simulink model "combinedTxRx_ADIDMA"  (R2017b)
settings: Solver=FixedStepDiscrete  StartTime=0.0  StopTime=10.0  RelTol=1e-3
InitFcn:
  | numHeaderBits = 16;
  | %numPreambleBits = 250;
  | AGCBarkerSymbols = 160+28;
  | EQTrainingSymbols = 250;
  | CRCGeneratorLag = 34; % CRCLen + 2
  | 
  | %% AGC Preamble
  | B13bipolar = [0 0 0 0 0 2 2 0 0 2 0 2];
  | rep = [B13bipolar, B13bipolar(1:4)];
  | AGCBarker = repmat(rep,1,10);
  | % Second preamble part
  | B11bipolar = [0 0 0 2 2 2 0 2  2 0 2];
  | TimingBarker = [B11bipolar,B11bipolar,B11bipolar,B11bipolar(1:6)];
  | PreambleBarkersInts = [AGCBarker, TimingBarker];
  | % Convert integer into their bit representation
  | PreambleBarkersBits = zeros(1,length(PreambleBarkersInts)*2);
  | PreambleBarkersBits(1:2:end) = (PreambleBarkersInts==2);
  | 
  | % Constants
  | % First preamble part
  | B13bipolar = [0 0 0 0 0 2 2 0 0 2 0 2];
  | rep = [B13bipolar, B13bipolar(1:4)];
  | AGCBarker = repmat(rep,1,10);
  | % Second preamble part
  | B11bipolar = [0 0 0 2 2 2 0 2  2 0 2];
  | TimingBarker = [B11bipolar,B11bipolar,B11bipolar(1:6)];
  | PreambleBarkersInts = [AGCBarker, TimingBarker];
  | % Convert integer into their bit representation
  | PreambleBarkersBits = false(1,length(PreambleBarkersInts)*2);
  | PreambleBarkersBits(1:2:end) = logical(PreambleBarkersInts==2);
  | pLen = uint16(length(PreambleBarkersBits));
  | 
  | 
  | %%%%%%%%%%%%%%%%%%%%%%%%%%
  | %% RX
  | %%%%%%%%%%%%%%%%%%%%%%%%%%
  | 
  | barker = comm.BarkerCode('SamplesPerFrame', 28, 'Length', 11);
  | seq = barker()+1;
  | M = 4;
  | hPSKModTrain   = comm.PSKModulator(M, ...
  |     'PhaseOffset',pi/4, ...
  |     'SymbolMapping','Binary');
  | xPreambleSeq = hPSKModTrain(seq);
  | 
  | 
  | %%%%%%%%%%%%
  | 
  | % AGC Preamble
  | reps = 5;
  | barker = comm.BarkerCode('SamplesPerFrame', 16, 'Length', 13);
  | seq = barker()+1;
  | %preamble = zeros(16*reps,1);
  | preambleFull = repmat(seq,reps,1);
  | rctFilt = comm.RaisedCosineTransmitFilter('FilterSpanInSymbols', 128,...
  | 'RolloffFactor',0.5,...
  | 'OutputSamplesPerSymbol',4);
  | preambleFullFilt = rctFilt(preambleFull);
  | 
  | %%%%%%%%%%%%
  | ... (+62 lines)
undefined symbols (not defined in the file or in its folder): j
libraries: simulink x20, dsphdlfiltering x20, hdlsllib x7, dspsigops x4, commseqgen3 x3, commdigbbndpm3 x3, commcrc2 x2, commcnvcod2 x2, commfilt2 x2, commsource2 x1, dspstat3 x1
(part 2 of 3)

== system combinedTxRx_ADIDMA/Combined TX and RX/Receiver HDL/Frame Recover/Equalization and Demodulation/DFE ==
  note: Generate training sequence when barker is found
  Trigger : Inport  PortDimensions=1
  data : Inport  Port=2  PortDimensions=1
      settings: SignalType=complex
  EQmu : Inport  Port=3
  DFE : Subsystem  mask{numFTaps=5, numBTaps=3, mu=0.01, refTap=2}
      mask prompts: numFTaps "Num Forward Taps"; numBTaps "Num Backward Taps"; mu "Step Size"; refTap "Reference Tap"
  Delay data so DFE can reset : Delay  DelayLength=1
  Delay ref so DFE can reset : Delay  DelayLength=1
  Equalizer : MATLAB Function  Commented=on  TreatAsAtomicUnit=on
  PN Sequence Generator : commseqgen3/PN Sequence Generator  poly='z^5 + z^3 + z^1 + 1'  ini_sta=[1 1 1 0 0]  outBitMaskSource=Dialog parameter  shift=0  outVarSiz=off  maxOutSizeMode=Dialog parameter  maxOutSize=[10 1]  Ts=-1  sampPerFrame=1  reset=on  bitPackedOutputs=on  outDataType=Smallest unsigned integer  numPackedBits=2  bitPackDataSigned=off  bitPackedOutDType=Smallest integer
      settings: SourceProductName=Communications System Toolbox
  Packeted To Unpacked : Subsystem
  QPSK Modulator Baseband : commdigbbndpm3/QPSK Modulator Baseband  InType=Bit  Enc=Binary  Ph=pi/4  outDtype=Fixed-point  outWordLen=16  outUDDataType=sfix(16)  outFracLenMode=User-defined  outFracLen=15  outDataTypeStr=fixdt(1,16,15)  outLastDataTypeStr=fixdt(1,16,15)
  Terminator1 : Terminator
  dataEQed : Outport
  start : Outport  Port=2
  wires:
  data/1 -> Delay data so DFE can reset/1
  PN Sequence Generator/1 -> Packeted To Unpacked/1(In1)
  Packeted To Unpacked/1(Out1) -> QPSK Modulator Baseband/1
  QPSK Modulator Baseband/1 -> Delay ref so DFE can reset/1
  DFE/3(start) -> start/1
  Trigger/1 -> DFE/1(reset), PN Sequence Generator/1
  DFE/2(err) -> Terminator1/1
  DFE/1(eqOut) -> dataEQed/1
  Delay data so DFE can reset/1 -> DFE/2(dataIn)
  Delay ref so DFE can reset/1 -> DFE/3(training)
  EQmu/1 -> DFE/4(EQmu)

== system combinedTxRx_ADIDMA/Combined TX and RX/Receiver HDL/Frame Recover/Frequency Recovery/Loop Filter ==
  note: This inflation is necessary
  note: Proportional-plus-Integrator Loop Filter,
      | Infinite DC Response to guarantee convergence
  e : Inport
  Add1 : Sum  RndMeth=Nearest  OutDataTypeStr=Inherit: Same as first input
  Add2 : Sum  OutDataTypeStr=Inherit: Same as first input
  Data Type Conversion : DataTypeConversion  OutDataTypeStr=fixdt(1,25,20)
  Delay : Delay  DelayLength=1
  Delay3 : Delay  DelayLength=1
  Delay4 : Delay  DelayLength=1
  K1 : Gain  Gain=K2  OutDataTypeStr=Inherit: Same as input
  K2 : Gain  Gain=K1  OutDataTypeStr=Inherit: Same as input
  Sum2 : Sum  OutDataTypeStr=Inherit: Same as first input
  v : Outport
  wires:
  K1/1 -> Sum2/1
  Add1/1 -> Sum2/2
  e/1 -> K2/1, K1/1
  K2/1 -> Delay/1, Add1/2
  Delay/1 -> Add1/1
  Sum2/1 -> Delay3/1
  Delay3/1 -> Add2/1
  Delay4/1 -> Add2/2
  Add2/1 -> Delay4/1, Data Type Conversion/1
  Data Type Conversion/1 -> v/1

== system combinedTxRx_ADIDMA/Combined TX and RX/Receiver HDL/Frame Recover/Frequency Recovery/Loop Filter Configurable ==
  note: This inflation is necessary
  note: Proportional-plus-Integrator Loop Filter,
      | Infinite DC Response to guarantee convergence
  e : Inport
  LoopBW : Inport  Port=2
  Add1 : Sum  RndMeth=Nearest  OutDataTypeStr=Inherit: Same as first input
  Add2 : Sum  OutDataTypeStr=Inherit: Same as first input
  Data Type Conversion : DataTypeConversion  OutDataTypeStr=fixdt(1,25,20)
  Delay : Delay  DelayLength=1
  Delay3 : Delay  DelayLength=1
  Delay4 : Delay  DelayLength=1
  Direct Lookup Table (n-D) : LookupNDDirect  NumberOfTableDimensions=1  Table=K1  DiagnosticForOutOfRangeInput=Error
  Direct Lookup Table (n-D)1 : LookupNDDirect  NumberOfTableDimensions=1  Table=K2  DiagnosticForOutOfRangeInput=Error
  Product : Product  OutDataTypeStr=Inherit: Same as first input
  Product1 : Product  OutDataTypeStr=Inherit: Same as first input
  Sum2 : Sum  OutDataTypeStr=Inherit: Same as first input
  v : Outport
  wires:
  Product/1 -> Sum2/1
  Add1/1 -> Sum2/2
  e/1 -> Product1/1, Product/1
  Product1/1 -> Delay/1, Add1/2
  Delay/1 -> Add1/1
  Sum2/1 -> Delay3/1
  Delay3/1 -> Add2/1
  Delay4/1 -> Add2/2
  Add2/1 -> Delay4/1, Data Type Conversion/1
  Data Type Conversion/1 -> v/1
  Direct Lookup Table (n-D)/1 -> Product/2
  Direct Lookup Table (n-D)1/1 -> Product1/2
  LoopBW/1 -> Direct Lookup Table (n-D)/1, Direct Lookup Table (n-D)1/1

== system combinedTxRx_ADIDMA/Combined TX and RX/Receiver HDL/Frame Recover/Frequency Recovery/Phase Shift FP ==
  note: Sign Comes from original
      | loop filter design
  In1 : Inport
  Phi : Inport  Port=2
  Cosine HDL Optimized : hdlsllib/Lookup Tables/Cosine HDL Optimized  OutputFormula=exp(j*2*pi*u)  NumDataPoints=256  TableDataTypeStr=fixdt(0,31,20)  SimulateLUTROMDelay=off
      settings: SourceProductName=HDL Coder  SourceProductBaseCode=HD
  Gain : Gain  Gain=-1/(2*pi)  ParamDataTypeStr=fixdt(1,25,20)  OutDataTypeStr=fixdt(1,16,12)  SaturateOnIntegerOverflow=on
  Product : Product  OutDataTypeStr=fixdt(1,16,13)  SaturateOnIntegerOverflow=on
  Out1 : Outport
  wires:
  Product/1 -> Out1/1
  Cosine HDL Optimized/1 -> Product/2
  In1/1 -> Product/1
  Phi/1 -> Gain/1
  Gain/1 -> Cosine HDL Optimized/1

== system combinedTxRx_ADIDMA/Combined TX and RX/Receiver HDL/Frame Recover/Gardner Timing Recovery/Gardner TED Blocks ==
  note: An input of 4 should not
      | happen unless the input is all zeros
  note: This is for QPSK and 4 SamplesPerSymbol ONLY
  data : Inport
  strobe : Inport  Port=2
  Add : Sum  OutDataTypeStr=fixdt(1,16,15)
  Check Only Strobe Condition : simulink/Logic and Bit Operations/Compare To Constant  relop===  const=uint8(1)  OutDataTypeStr=boolean
  Complex to Real-Imag : ComplexToRealImag
  Constant : Constant  Value=0  OutDataTypeStr=Inherit: Inherit via back propagation  SampleTime=-1
  Display : Display
  Imag Error : Subsystem
  Logical Operator : Logic  AllPortsSameDT=off  OutDataTypeStr=boolean
  Map [0,1,2,3,4] to [0,1,2,2,2] : LookupNDDirect  NumberOfTableDimensions=1  Table=[0 1 2 2 2]  DiagnosticForOutOfRangeInput=Error  TableDataTypeStr=uint8
  Real Error : Subsystem
  Strobe Buffer1 : simulink/Discrete/Tapped Delay  vinit=0.0  samptime=-1  NumDelays=samplesPerSymbol-1  DelayOrder=Oldest  includeCurrent=on
  Sum of Elements1 : Sum  Inputs=+  OutDataTypeStr=int8
  Switch : Switch  Criteria=u2 ~= 0  SaturateOnIntegerOverflow=on
  e : Outport
  wires:
  Switch/1 -> e/1
  strobe/1 -> Strobe Buffer1/1, Logical Operator/2
  Complex to Real-Imag/2 -> Imag Error/1(data)
  Sum of Elements1/1 -> Display/1, Check Only Strobe Condition/1, Map [0,1,2,3,4] to [0,1,2,2,2]/1
  Check Only Strobe Condition/1 -> Logical Operator/1
  Constant/1 -> Switch/3
  Complex to Real-Imag/1 -> Real Error/1(data)
  data/1 -> Complex to Real-Imag/1
  Map [0,1,2,3,4] to [0,1,2,2,2]/1 -> Imag Error/2(strobe sum), Real Error/2(strobe sum)
  Strobe Buffer1/1 -> Sum of Elements1/1
  Real Error/1(Out1) -> Add/1
  Imag Error/1(Out1) -> Add/2
  Add/1 -> Switch/1
  Logical Operator/1 -> Switch/2

== system combinedTxRx_ADIDMA/Combined TX and RX/Receiver HDL/Frame Recover/Gardner Timing Recovery/InterpControl_Blocks1 ==
  note: e<<1/SPS
  note: Mu is always positive
  e : Inport
  1/SPS1 : Constant  Value=fi(1/samplesPerSymbol,0,2,2)  OutDataTypeStr=fixdt(0,2,2)  SampleTime=-1
  Add1 : Sum  OutDataTypeStr=fixdt(0,16,16)
  Calculate New mu : Subsystem
  Display{,1..3} (4 alike) : Display
  Mod 1 : Subsystem
  NCOCounter State : Delay  DelayLength=1  InitialCondition=0
  Subtract1 : Sum  Inputs=-+  OutDataTypeStr=Inherit: Same as first input
  Update mu on strobe : Switch  Criteria=u2 > Threshold
  saved mu : Delay  DelayLength=1
  strobe == W>NCOCounter : RelationalOperator  Operator=>  OutDataTypeStr=boolean  RndMeth=Nearest
  strobe : Outport
  mu : Outport  Port=2
  wires:
  strobe == W>NCOCounter/1 -> Update mu on strobe/2, strobe/1
  Update mu on strobe/1 -> Display3/1, mu/1, saved mu/1
  saved mu/1 -> Update mu on strobe/3
  Calculate New mu/1(mu) -> Display/1, Update mu on strobe/1
  e/1 -> Add1/1
  NCOCounter State/1 -> Subtract1/2, Display1/1, strobe == W>NCOCounter/2, Calculate New mu/2(NCOCounter)
  Subtract1/1 -> Mod 1/1(In1)
  Mod 1/1(Out1) -> NCOCounter State/1
  1/SPS1/1 -> Add1/2
  Add1/1 -> Calculate New mu/1(W), strobe == W>NCOCounter/1, Display2/1, Subtract1/1

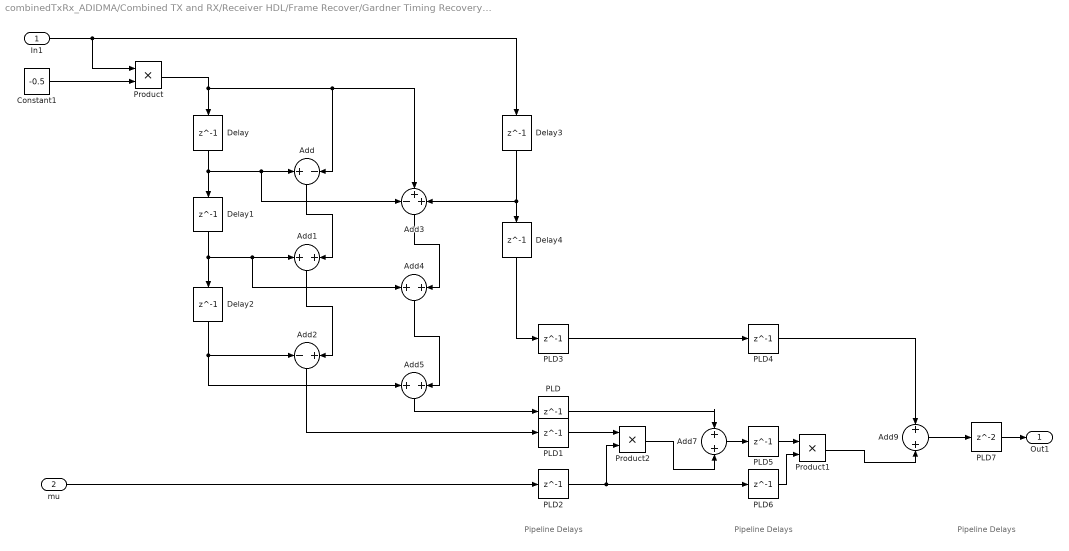
== system combinedTxRx_ADIDMA/Combined TX and RX/Receiver HDL/Frame Recover/Gardner Timing Recovery/Interpolator ==
  note: Pipeline Delays
  note: Pipeline Delays
  note: Pipeline Delays
  In1 : Inport
  mu : Inport  Port=2
  Add : Sum  Inputs=+-  OutDataTypeStr=Inherit: Same as first input
  Add{1,4..5,7} (4 alike) : Sum
  Add2 : Sum  Inputs=-+
  Add3 : Sum  Inputs=-++
  Add9 : Sum  OutDataTypeStr=fixdt(1,16,10)
  Constant1 : Constant  Value=-0.5  OutDataTypeStr=fixdt(1,2,2)  SampleTime=-1
  Delay{,1..4} (5 alike) : Delay  DelayLength=1
  PLD{,1..6} (7 alike) : Delay  DelayLength=1
  PLD7 : Delay
  Product : Product  OutDataTypeStr=fixdt(1,16,14)
  Product1 : Product
  Product2 : Product  OutDataTypeStr=fixdt(1,16,10)
  Out1 : Outport
  wires:
  In1/1 -> Delay3/1, Product/1
  Product/1 -> Add3/2, Add/2, Delay/1
  Delay/1 -> Add3/1, Add/1, Delay1/1
  Delay1/1 -> Add4/1, Add1/1, Delay2/1
  Add/1 -> Add1/2
  Delay2/1 -> Add5/1, Add2/1
  Add1/1 -> Add2/2
  Add3/1 -> Add4/2
  Add4/1 -> Add5/2
  Add2/1 -> PLD1/1
  mu/1 -> PLD2/1
  Add5/1 -> PLD/1
  Product2/1 -> Add7/2
  Add9/1 -> PLD7/1
  Delay3/1 -> Delay4/1, Add3/3
  Delay4/1 -> PLD3/1
  Add7/1 -> PLD5/1
  Product1/1 -> Add9/2
  Constant1/1 -> Product/2
  PLD/1 -> Add7/1
  PLD1/1 -> Product2/1
  PLD2/1 -> Product2/2, PLD6/1
  PLD3/1 -> PLD4/1
  PLD4/1 -> Add9/1
  PLD5/1 -> Product1/1
  PLD6/1 -> Product1/2
  PLD7/1 -> Out1/1

== system combinedTxRx_ADIDMA/Combined TX and RX/Receiver HDL/Frame Recover/Gardner Timing Recovery/LoopFilter1 ==
  e : Inport
  Delay1 : Delay  DelayLength=1
  Delay2 : Delay  DelayLength=1
  Proportional Gain : Gain  Gain=fi(ProportionalGain,1,16,15)  OutDataTypeStr=fixdt(1,16,24)
  v : Outport
  wires:
  e/1 -> Delay2/1
  Proportional Gain/1 -> Delay1/1
  Delay2/1 -> Proportional Gain/1
  Delay1/1 -> v/1

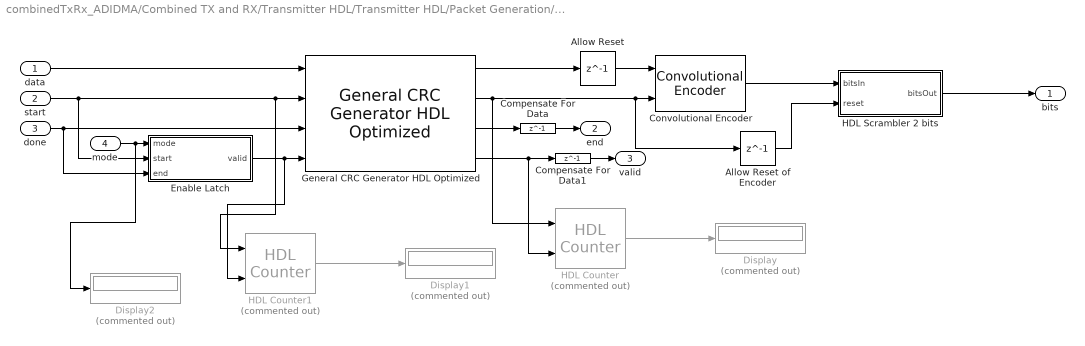
== system combinedTxRx_ADIDMA/Combined TX and RX/Transmitter HDL/Transmitter HDL/Packet Generation/Payload ==
  data : Inport
  start : Inport  Port=2
  done : Inport  Port=3
  mode : Inport  Port=4
  Allow Reset : Delay  DelayLength=1
  Allow Reset of Encoder : Delay  DelayLength=1
  Compensate For Data : Delay  DelayLength=1
  Compensate For Data1 : Delay  DelayLength=1
  Convolutional Encoder : commcnvcod2/Convolutional Encoder  trellis=poly2trellis(7, [171 133])  opMode=Reset on nonzero input via port  DelayedResetAction=on  hasIniStPort=off  hasFinStPort=off  usePuncVector=off  punctureVector=[1; 1; 0; 1; 0; 1]  reset=Unused parameter value
      settings: SourceProductName=Communications System Toolbox  SourceProductBaseCode=CM
  Display : Display  Commented=on
  Display1 : Display  Commented=on
  Display2 : Display  Commented=on
  Enable Latch : Subsystem
  General CRC Generator HDL Optimized : commcrc2/General CRC Generator HDL Optimized  Polynomial=[1 0 0 0 0 0 1 0 0 1 1 0 0 0 0 0 1 0 0 0 1 1 1 0 1 1 0 1 1 0 1 1 1]  InitialState=0  DirectMethod=off  ReflectInput=off  ReflectCRCChecksum=off  FinalXORValue=0  SimulateUsing=Code generation
      settings: SourceProductName=Communications System Toolbox  SourceProductBaseCode=CM
  HDL Counter : hdlsllib/Sources/HDL Counter  Commented=on  CountType=Count limited  CountInit=0  CountStep=1  CountMax=1e4  CountFromType=Initial value  CountFrom=0  CountResetPort=on  CountLoadPort=off  CountEnbPort=on  CountDirPort=off  CountDataType=Unsigned  CountWordLen=16  CountFracLen=0  CountSampTime=1
      settings: SourceProductBaseCode=HD
  HDL Counter1 : hdlsllib/Sources/HDL Counter  Commented=on  CountType=Count limited  CountInit=0  CountStep=1  CountMax=1e4  CountFromType=Initial value  CountFrom=0  CountResetPort=on  CountLoadPort=off  CountEnbPort=on  CountDirPort=off  CountDataType=Unsigned  CountWordLen=16  CountFracLen=0  CountSampTime=1
      settings: SourceProductBaseCode=HD
  HDL Scrambler 2 bits : Subsystem  mask{poly=[1 1 0 1 0 1 0 1], init_state=[0 1 0 0 0 1 0]}
      mask prompts: poly "Polynomial"; init_state "Initial State"
  bits : Outport
  end : Outport  Port=2
  valid : Outport  Port=3
  wires:
  General CRC Generator HDL Optimized/1 -> Allow Reset/1
  data/1 -> General CRC Generator HDL Optimized/1
  start/1 -> Enable Latch/2(start), HDL Counter1/1, General CRC Generator HDL Optimized/2
  General CRC Generator HDL Optimized/4 -> HDL Counter/2, Compensate For Data1/1
  done/1 -> Enable Latch/3(end), General CRC Generator HDL Optimized/3
  mode/1 -> Display2/1, Enable Latch/1(mode)
  Convolutional Encoder/1 -> HDL Scrambler 2 bits/1(bitsIn)
  General CRC Generator HDL Optimized/2 -> HDL Counter/1, Allow Reset of Encoder/1, Convolutional Encoder/2
  HDL Scrambler 2 bits/1(bitsOut) -> bits/1
  Enable Latch/1(valid) -> HDL Counter1/2, General CRC Generator HDL Optimized/4
  Allow Reset/1 -> Convolutional Encoder/1
  Allow Reset of Encoder/1 -> HDL Scrambler 2 bits/2(reset)
  HDL Counter/1 -> Display/1
  HDL Counter1/1 -> Display1/1
  Compensate For Data/1 -> end/1
  Compensate For Data1/1 -> valid/1
  General CRC Generator HDL Optimized/3 -> Compensate For Data/1

== system combinedTxRx_ADIDMA/Combined TX and RX/Transmitter HDL/Transmitter HDL/Packet Generation/Preamble ==
  reset : Inport
  Barker Even : LookupNDDirect  NumberOfTableDimensions=1  Table=[PreambleBarkersBits(4:2:end),false(1,400)]  DiagnosticForOutOfRangeInput=Error  TableDataTypeStr=boolean
  Barker Odd : LookupNDDirect  NumberOfTableDimensions=1  Table=[PreambleBarkersBits(3:2:end-1),false(1,400)]  DiagnosticForOutOfRangeInput=Error  TableDataTypeStr=boolean
  Delay{,1..3} (4 alike) : Delay  DelayLength=1
  Enable at end of barker : simulink/Logic and Bit Operations/Compare To Constant  relop=<  const=pLen/2-1  OutDataTypeStr=boolean
  HDL Counter : hdlsllib/Sources/HDL Counter  CountType=Count limited  CountInit=0  CountStep=1  CountMax=pLen/2-2+400  CountFromType=Initial value  CountFrom=0  CountResetPort=on  CountLoadPort=off  CountEnbPort=off  CountDirPort=off  CountDataType=Unsigned  CountWordLen=16  CountFracLen=0  CountSampTime=1
      settings: SourceProductBaseCode=HD
  PN Sequence For EQ : commseqgen3/PN Sequence Generator  poly='z^5 + z^3 + z^1 + 1'  ini_sta=[1 1 1 0 0]  outBitMaskSource=Dialog parameter  shift=0  outVarSiz=off  maxOutSizeMode=Dialog parameter  maxOutSize=[10 1]  Ts=-1  sampPerFrame=1  reset=on  bitPackedOutputs=on  outDataType=double  numPackedBits=2  bitPackDataSigned=off  bitPackedOutDType=Smallest integer
      settings: SourceProductName=Communications System Toolbox
  Reset When Barkers Are Done : simulink/Logic and Bit Operations/Compare To Constant  relop===  const=pLen/2-1  OutDataTypeStr=boolean
  Switch1 : Switch  Threshold=1
  Unpack1 : Subsystem
  Vector Concatenate1 : Concatenate
  Out1 : Outport
  wires:
  reset/1 -> HDL Counter/1
  Barker Odd/1 -> Vector Concatenate1/1
  Barker Even/1 -> Vector Concatenate1/2
  PN Sequence For EQ/1 -> Unpack1/1(In1)
  Switch1/1 -> Out1/1
  Reset When Barkers Are Done/1 -> PN Sequence For EQ/1
  HDL Counter/1 -> Delay/1
  Delay/1 -> Enable at end of barker/1, Reset When Barkers Are Done/1, Barker Even/1, Barker Odd/1
  Vector Concatenate1/1 -> Delay1/1
  Enable at end of barker/1 -> Delay2/1
  Unpack1/1(Out1) -> Delay3/1
  Delay1/1 -> Switch1/1
  Delay2/1 -> Switch1/2
  Delay3/1 -> Switch1/3

== system combinedTxRx_ADIDMA/Combined TX and RX/Transmitter HDL/Transmitter HDL/Packet Generation/Random Data ==
  In1 : Inport
  Random Data Gen : commseqgen3/PN Sequence Generator  poly='z^3 + z^2 + 1'  ini_sta=[0 0 1]  outBitMaskSource=Dialog parameter  shift=0  outVarSiz=off  maxOutSizeMode=Dialog parameter  maxOutSize=[10 1]  Ts=-1  sampPerFrame=1  reset=on  bitPackedOutputs=on  outDataType=double  numPackedBits=2  bitPackDataSigned=off  bitPackedOutDType=Smallest integer
      settings: SourceProductName=Communications System Toolbox
  Unpack : Subsystem
  Out1 : Outport
  wires:
  In1/1 -> Random Data Gen/1
  Unpack/1(Out1) -> Out1/1
  Random Data Gen/1 -> Unpack/1(In1)

== system combinedTxRx_ADIDMA/Combined TX and RX/Receiver HDL/Frame Recover/Barker Locate/Measure Phase Ambiguity/Find Max and Set Output Shift ==
  In1 : Inport
  In2 : Inport  Port=2
  In4 : Inport  Port=3
  In5 : Inport  Port=4
  Enable : EnablePort
  Complex to Real-Imag{,1..3} (4 alike) : ComplexToRealImag  Output=Imag
  Direct Lookup Table (n-D) : LookupNDDirect  NumberOfTableDimensions=1  Table=exp(-(0:pi/2:(pi*3/2)) .* 1i).'  DiagnosticForOutOfRangeInput=Error  TableDataTypeStr=fixdt(1,16,13)
  Display : Display
  Display1 : Display
  Maximum : dspstat3/Maximum  operation=maximum  fcn=Index  indexBase=Zero  operateOver=Each column  Dimension=1  InputProcessing=Columns as channels (frame based)  reset=None  roiEnable=off  roiType=Rectangles  roiPortion=Entire ROI  roiOutput=Individual statistics for each ROI  roiFlag=off  roundingMode=Floor  overflowMode=off  accumDataTypeStr=Inherit: Same as product output  accumLastDataTypeStr=Inherit: Same as product output
  Vector Concatenate : Concatenate  NumInputs=4
  Vector Concatenate1 : Concatenate  NumInputs=4
  Out1 : Outport  InitialOutput=0
  wires:
  Direct Lookup Table (n-D)/1 -> Out1/1
  In4/1 -> Vector Concatenate1/3, Complex to Real-Imag2/1
  In2/1 -> Vector Concatenate1/2, Complex to Real-Imag1/1
  In5/1 -> Vector Concatenate1/4, Complex to Real-Imag3/1
  In1/1 -> Vector Concatenate1/1, Complex to Real-Imag/1
  Maximum/1 -> Direct Lookup Table (n-D)/1
  Vector Concatenate/1 -> Display/1, Maximum/1
  Vector Concatenate1/1 -> Display1/1
  Complex to Real-Imag1/1 -> Vector Concatenate/2
  Complex to Real-Imag3/1 -> Vector Concatenate/4
  Complex to Real-Imag2/1 -> Vector Concatenate/3
  Complex to Real-Imag/1 -> Vector Concatenate/1

== system combinedTxRx_ADIDMA/Combined TX and RX/Receiver HDL/Frame Recover/Barker Locate/Measure Phase Ambiguity/HDL Opt Complex FIR4 ==
  In1 : Inport
  validIn : Inport  Port=2
  Add : Sum  Inputs=+-  AccumDataTypeStr=fixdt(1,16,0)
  Complex to Real-Imag : ComplexToRealImag
  Discrete FIR Filter HDL Optimized : dsphdlfiltering/Discrete FIR Filter HDL Optimized  Numerator=real(Taps)  Sharing=off  SharingFactor=2  SimulateUsing=Code generation  roundingMode=Floor  overflowMode=off  CoefficientsDataTypeStr=Inherit: Same word length as input  CoefficientsMin=[]  CoefficientsMax=[]  OutputDataTypeStr=fixdt(1,16,0)  OutputMin=[]  OutputMax=[]  ValidInPort=on  ReadyPort=off
      settings: SourceProductName=DSP System Toolbox  SourceProductBaseCode=DS
  Discrete FIR Filter HDL Optimized1 : dsphdlfiltering/Discrete FIR Filter HDL Optimized  Numerator=imag(Taps)  Sharing=off  SharingFactor=2  SimulateUsing=Code generation  roundingMode=Floor  overflowMode=off  CoefficientsDataTypeStr=Inherit: Same word length as input  CoefficientsMin=[]  CoefficientsMax=[]  OutputDataTypeStr=fixdt(1,16,0)  OutputMin=[]  OutputMax=[]  ValidInPort=on  ReadyPort=off
      settings: SourceProductName=DSP System Toolbox  SourceProductBaseCode=DS
  Discrete FIR Filter HDL Optimized2 : dsphdlfiltering/Discrete FIR Filter HDL Optimized  Numerator=real(Taps)  Sharing=off  SharingFactor=2  SimulateUsing=Code generation  roundingMode=Floor  overflowMode=off  CoefficientsDataTypeStr=Inherit: Same word length as input  CoefficientsMin=[]  CoefficientsMax=[]  OutputDataTypeStr=fixdt(1,16,0)  OutputMin=[]  OutputMax=[]  ValidInPort=on  ReadyPort=off
      settings: SourceProductName=DSP System Toolbox  SourceProductBaseCode=DS
  Discrete FIR Filter HDL Optimized3 : dsphdlfiltering/Discrete FIR Filter HDL Optimized  Numerator=imag(Taps)  Sharing=off  SharingFactor=2  SimulateUsing=Code generation  roundingMode=Floor  overflowMode=off  CoefficientsDataTypeStr=Inherit: Same word length as input  CoefficientsMin=[]  CoefficientsMax=[]  OutputDataTypeStr=fixdt(1,16,0)  OutputMin=[]  OutputMax=[]  ValidInPort=on  ReadyPort=off
      settings: SourceProductName=DSP System Toolbox  SourceProductBaseCode=DS
  Logical Operator : Logic  Inputs=4  AllPortsSameDT=off  OutDataTypeStr=boolean
  Real-Imag to Complex : RealImagToComplex
  Subtract : Sum  OutDataTypeStr=int16
  Out1 : Outport
  validOut : Outport  Port=2
  wires:
  Discrete FIR Filter HDL Optimized/1 -> Add/1
  Logical Operator/1 -> validOut/1
  Discrete FIR Filter HDL Optimized/2 -> Logical Operator/1
  Discrete FIR Filter HDL Optimized1/2 -> Logical Operator/2
  Discrete FIR Filter HDL Optimized1/1 -> Add/2
  validIn/1 -> Discrete FIR Filter HDL Optimized3/2, Discrete FIR Filter HDL Optimized2/2, Discrete FIR Filter HDL Optimized1/2, Discrete FIR Filter HDL Optimized/2
  In1/1 -> Complex to Real-Imag/1
  Complex to Real-Imag/1 -> Discrete FIR Filter HDL Optimized3/1, Discrete FIR Filter HDL Optimized/1
  Discrete FIR Filter HDL Optimized2/2 -> Logical Operator/3
  Discrete FIR Filter HDL Optimized3/2 -> Logical Operator/4
  Complex to Real-Imag/2 -> Discrete FIR Filter HDL Optimized2/1, Discrete FIR Filter HDL Optimized1/1
  Discrete FIR Filter HDL Optimized2/1 -> Subtract/1
  Discrete FIR Filter HDL Optimized3/1 -> Subtract/2
  Real-Imag to Complex/1 -> Out1/1
  Subtract/1 -> Real-Imag to Complex/2
  Add/1 -> Real-Imag to Complex/1

== system combinedTxRx_ADIDMA/Combined TX and RX/Receiver HDL/Frame Recover/Barker Locate/Measure Phase Ambiguity/HDL Opt Complex FIR5 ==
  In1 : Inport
  validIn : Inport  Port=2
  Add : Sum  Inputs=+-  AccumDataTypeStr=fixdt(1,16,0)
  Complex to Real-Imag : ComplexToRealImag
  Discrete FIR Filter HDL Optimized : dsphdlfiltering/Discrete FIR Filter HDL Optimized  Numerator=real(Taps)  Sharing=off  SharingFactor=2  SimulateUsing=Code generation  roundingMode=Floor  overflowMode=off  CoefficientsDataTypeStr=Inherit: Same word length as input  CoefficientsMin=[]  CoefficientsMax=[]  OutputDataTypeStr=fixdt(1,16,0)  OutputMin=[]  OutputMax=[]  ValidInPort=on  ReadyPort=off
      settings: SourceProductName=DSP System Toolbox  SourceProductBaseCode=DS
  Discrete FIR Filter HDL Optimized1 : dsphdlfiltering/Discrete FIR Filter HDL Optimized  Numerator=imag(Taps)  Sharing=off  SharingFactor=2  SimulateUsing=Code generation  roundingMode=Floor  overflowMode=off  CoefficientsDataTypeStr=Inherit: Same word length as input  CoefficientsMin=[]  CoefficientsMax=[]  OutputDataTypeStr=fixdt(1,16,0)  OutputMin=[]  OutputMax=[]  ValidInPort=on  ReadyPort=off
      settings: SourceProductName=DSP System Toolbox  SourceProductBaseCode=DS
  Discrete FIR Filter HDL Optimized2 : dsphdlfiltering/Discrete FIR Filter HDL Optimized  Numerator=real(Taps)  Sharing=off  SharingFactor=2  SimulateUsing=Code generation  roundingMode=Floor  overflowMode=off  CoefficientsDataTypeStr=Inherit: Same word length as input  CoefficientsMin=[]  CoefficientsMax=[]  OutputDataTypeStr=fixdt(1,16,0)  OutputMin=[]  OutputMax=[]  ValidInPort=on  ReadyPort=off
      settings: SourceProductName=DSP System Toolbox  SourceProductBaseCode=DS
  Discrete FIR Filter HDL Optimized3 : dsphdlfiltering/Discrete FIR Filter HDL Optimized  Numerator=imag(Taps)  Sharing=off  SharingFactor=2  SimulateUsing=Code generation  roundingMode=Floor  overflowMode=off  CoefficientsDataTypeStr=Inherit: Same word length as input  CoefficientsMin=[]  CoefficientsMax=[]  OutputDataTypeStr=fixdt(1,16,0)  OutputMin=[]  OutputMax=[]  ValidInPort=on  ReadyPort=off
      settings: SourceProductName=DSP System Toolbox  SourceProductBaseCode=DS
  Logical Operator : Logic  Inputs=4  AllPortsSameDT=off  OutDataTypeStr=boolean
  Real-Imag to Complex : RealImagToComplex
  Subtract : Sum  OutDataTypeStr=int16
  Out1 : Outport
  validOut : Outport  Port=2
  wires:
  Discrete FIR Filter HDL Optimized/1 -> Add/1
  Logical Operator/1 -> validOut/1
  Discrete FIR Filter HDL Optimized/2 -> Logical Operator/1
  Discrete FIR Filter HDL Optimized1/2 -> Logical Operator/2
  Discrete FIR Filter HDL Optimized1/1 -> Add/2
  validIn/1 -> Discrete FIR Filter HDL Optimized3/2, Discrete FIR Filter HDL Optimized2/2, Discrete FIR Filter HDL Optimized1/2, Discrete FIR Filter HDL Optimized/2
  In1/1 -> Complex to Real-Imag/1
  Complex to Real-Imag/1 -> Discrete FIR Filter HDL Optimized3/1, Discrete FIR Filter HDL Optimized/1
  Discrete FIR Filter HDL Optimized2/2 -> Logical Operator/3
  Discrete FIR Filter HDL Optimized3/2 -> Logical Operator/4
  Complex to Real-Imag/2 -> Discrete FIR Filter HDL Optimized2/1, Discrete FIR Filter HDL Optimized1/1
  Discrete FIR Filter HDL Optimized2/1 -> Subtract/1
  Discrete FIR Filter HDL Optimized3/1 -> Subtract/2
  Real-Imag to Complex/1 -> Out1/1
  Subtract/1 -> Real-Imag to Complex/2
  Add/1 -> Real-Imag to Complex/1

== system combinedTxRx_ADIDMA/Combined TX and RX/Receiver HDL/Frame Recover/Barker Locate/Measure Phase Ambiguity/HDL Opt Complex FIR6 ==
  In1 : Inport
  validIn : Inport  Port=2
  Add : Sum  Inputs=+-  AccumDataTypeStr=fixdt(1,16,0)
  Complex to Real-Imag : ComplexToRealImag
  Discrete FIR Filter HDL Optimized : dsphdlfiltering/Discrete FIR Filter HDL Optimized  Numerator=real(Taps)  Sharing=off  SharingFactor=2  SimulateUsing=Code generation  roundingMode=Floor  overflowMode=off  CoefficientsDataTypeStr=Inherit: Same word length as input  CoefficientsMin=[]  CoefficientsMax=[]  OutputDataTypeStr=fixdt(1,16,0)  OutputMin=[]  OutputMax=[]  ValidInPort=on  ReadyPort=off
      settings: SourceProductName=DSP System Toolbox  SourceProductBaseCode=DS
  Discrete FIR Filter HDL Optimized1 : dsphdlfiltering/Discrete FIR Filter HDL Optimized  Numerator=imag(Taps)  Sharing=off  SharingFactor=2  SimulateUsing=Code generation  roundingMode=Floor  overflowMode=off  CoefficientsDataTypeStr=Inherit: Same word length as input  CoefficientsMin=[]  CoefficientsMax=[]  OutputDataTypeStr=fixdt(1,16,0)  OutputMin=[]  OutputMax=[]  ValidInPort=on  ReadyPort=off
      settings: SourceProductName=DSP System Toolbox  SourceProductBaseCode=DS
  Discrete FIR Filter HDL Optimized2 : dsphdlfiltering/Discrete FIR Filter HDL Optimized  Numerator=real(Taps)  Sharing=off  SharingFactor=2  SimulateUsing=Code generation  roundingMode=Floor  overflowMode=off  CoefficientsDataTypeStr=Inherit: Same word length as input  CoefficientsMin=[]  CoefficientsMax=[]  OutputDataTypeStr=fixdt(1,16,0)  OutputMin=[]  OutputMax=[]  ValidInPort=on  ReadyPort=off
      settings: SourceProductName=DSP System Toolbox  SourceProductBaseCode=DS
  Discrete FIR Filter HDL Optimized3 : dsphdlfiltering/Discrete FIR Filter HDL Optimized  Numerator=imag(Taps)  Sharing=off  SharingFactor=2  SimulateUsing=Code generation  roundingMode=Floor  overflowMode=off  CoefficientsDataTypeStr=Inherit: Same word length as input  CoefficientsMin=[]  CoefficientsMax=[]  OutputDataTypeStr=fixdt(1,16,0)  OutputMin=[]  OutputMax=[]  ValidInPort=on  ReadyPort=off
      settings: SourceProductName=DSP System Toolbox  SourceProductBaseCode=DS
  Logical Operator : Logic  Inputs=4  AllPortsSameDT=off  OutDataTypeStr=boolean
  Real-Imag to Complex : RealImagToComplex
  Subtract : Sum  OutDataTypeStr=int16
  Out1 : Outport
  validOut : Outport  Port=2
  wires:
  Discrete FIR Filter HDL Optimized/1 -> Add/1
  Logical Operator/1 -> validOut/1
  Discrete FIR Filter HDL Optimized/2 -> Logical Operator/1
  Discrete FIR Filter HDL Optimized1/2 -> Logical Operator/2
  Discrete FIR Filter HDL Optimized1/1 -> Add/2
  validIn/1 -> Discrete FIR Filter HDL Optimized3/2, Discrete FIR Filter HDL Optimized2/2, Discrete FIR Filter HDL Optimized1/2, Discrete FIR Filter HDL Optimized/2
  In1/1 -> Complex to Real-Imag/1
  Complex to Real-Imag/1 -> Discrete FIR Filter HDL Optimized3/1, Discrete FIR Filter HDL Optimized/1
  Discrete FIR Filter HDL Optimized2/2 -> Logical Operator/3
  Discrete FIR Filter HDL Optimized3/2 -> Logical Operator/4
  Complex to Real-Imag/2 -> Discrete FIR Filter HDL Optimized2/1, Discrete FIR Filter HDL Optimized1/1
  Discrete FIR Filter HDL Optimized2/1 -> Subtract/1
  Discrete FIR Filter HDL Optimized3/1 -> Subtract/2
  Real-Imag to Complex/1 -> Out1/1
  Subtract/1 -> Real-Imag to Complex/2
  Add/1 -> Real-Imag to Complex/1

== system combinedTxRx_ADIDMA/Combined TX and RX/Receiver HDL/Frame Recover/Barker Locate/Measure Phase Ambiguity/HDL Opt Complex FIR7 ==
  In1 : Inport
  validIn : Inport  Port=2
  Add : Sum  Inputs=+-  AccumDataTypeStr=fixdt(1,16,0)
  Complex to Real-Imag : ComplexToRealImag
  Discrete FIR Filter HDL Optimized : dsphdlfiltering/Discrete FIR Filter HDL Optimized  Numerator=real(Taps)  Sharing=off  SharingFactor=2  SimulateUsing=Code generation  roundingMode=Floor  overflowMode=off  CoefficientsDataTypeStr=Inherit: Same word length as input  CoefficientsMin=[]  CoefficientsMax=[]  OutputDataTypeStr=fixdt(1,16,0)  OutputMin=[]  OutputMax=[]  ValidInPort=on  ReadyPort=off
      settings: SourceProductName=DSP System Toolbox  SourceProductBaseCode=DS
  Discrete FIR Filter HDL Optimized1 : dsphdlfiltering/Discrete FIR Filter HDL Optimized  Numerator=imag(Taps)  Sharing=off  SharingFactor=2  SimulateUsing=Code generation  roundingMode=Floor  overflowMode=off  CoefficientsDataTypeStr=Inherit: Same word length as input  CoefficientsMin=[]  CoefficientsMax=[]  OutputDataTypeStr=fixdt(1,16,0)  OutputMin=[]  OutputMax=[]  ValidInPort=on  ReadyPort=off
      settings: SourceProductName=DSP System Toolbox  SourceProductBaseCode=DS
  Discrete FIR Filter HDL Optimized2 : dsphdlfiltering/Discrete FIR Filter HDL Optimized  Numerator=real(Taps)  Sharing=off  SharingFactor=2  SimulateUsing=Code generation  roundingMode=Floor  overflowMode=off  CoefficientsDataTypeStr=Inherit: Same word length as input  CoefficientsMin=[]  CoefficientsMax=[]  OutputDataTypeStr=fixdt(1,16,0)  OutputMin=[]  OutputMax=[]  ValidInPort=on  ReadyPort=off
      settings: SourceProductName=DSP System Toolbox  SourceProductBaseCode=DS
  Discrete FIR Filter HDL Optimized3 : dsphdlfiltering/Discrete FIR Filter HDL Optimized  Numerator=imag(Taps)  Sharing=off  SharingFactor=2  SimulateUsing=Code generation  roundingMode=Floor  overflowMode=off  CoefficientsDataTypeStr=Inherit: Same word length as input  CoefficientsMin=[]  CoefficientsMax=[]  OutputDataTypeStr=fixdt(1,16,0)  OutputMin=[]  OutputMax=[]  ValidInPort=on  ReadyPort=off
      settings: SourceProductName=DSP System Toolbox  SourceProductBaseCode=DS
  Logical Operator : Logic  Inputs=4  AllPortsSameDT=off  OutDataTypeStr=boolean
  Real-Imag to Complex : RealImagToComplex
  Subtract : Sum  OutDataTypeStr=int16
  Out1 : Outport
  validOut : Outport  Port=2
  wires:
  Discrete FIR Filter HDL Optimized/1 -> Add/1
  Logical Operator/1 -> validOut/1
  Discrete FIR Filter HDL Optimized/2 -> Logical Operator/1
  Discrete FIR Filter HDL Optimized1/2 -> Logical Operator/2
  Discrete FIR Filter HDL Optimized1/1 -> Add/2
  validIn/1 -> Discrete FIR Filter HDL Optimized3/2, Discrete FIR Filter HDL Optimized2/2, Discrete FIR Filter HDL Optimized1/2, Discrete FIR Filter HDL Optimized/2
  In1/1 -> Complex to Real-Imag/1
  Complex to Real-Imag/1 -> Discrete FIR Filter HDL Optimized3/1, Discrete FIR Filter HDL Optimized/1
  Discrete FIR Filter HDL Optimized2/2 -> Logical Operator/3
  Discrete FIR Filter HDL Optimized3/2 -> Logical Operator/4
  Complex to Real-Imag/2 -> Discrete FIR Filter HDL Optimized2/1, Discrete FIR Filter HDL Optimized1/1
  Discrete FIR Filter HDL Optimized2/1 -> Subtract/1
  Discrete FIR Filter HDL Optimized3/1 -> Subtract/2
  Real-Imag to Complex/1 -> Out1/1
  Subtract/1 -> Real-Imag to Complex/2
  Add/1 -> Real-Imag to Complex/1

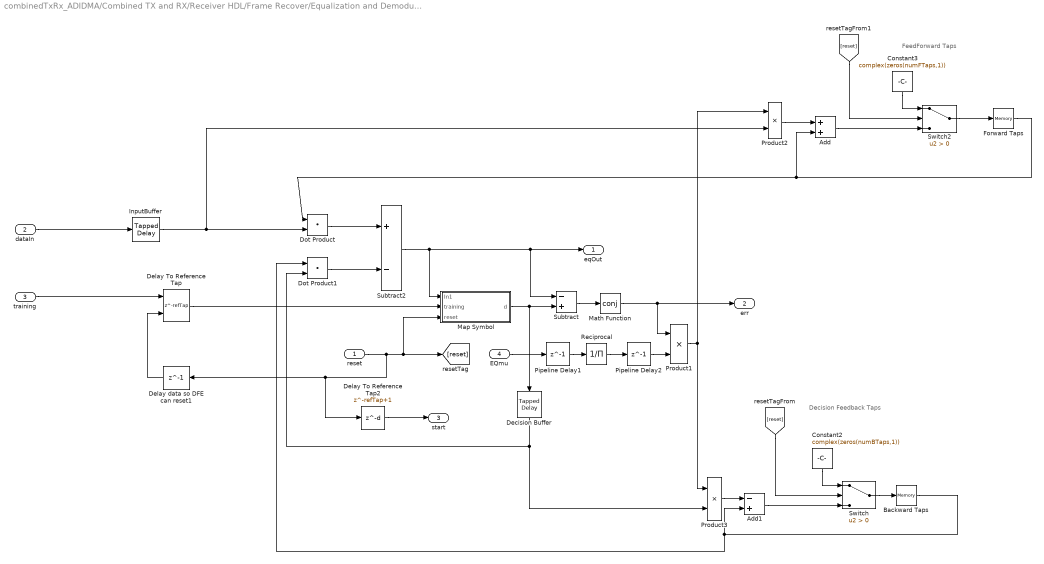
== system combinedTxRx_ADIDMA/Combined TX and RX/Receiver HDL/Frame Recover/Equalization and Demodulation/DFE/DFE ==
  note: FeedForward Taps
  note: Decision Feedback Taps
  reset : Inport
  dataIn : Inport  Port=2  OutDataTypeStr=fixdt(1,16,14)
  training : Inport  Port=3  OutDataTypeStr=fixdt(1,16,15)
  EQmu : Inport  Port=4
  Add : Sum  OutDataTypeStr=fixdt(1,16,14)
  Add1 : Sum  Inputs=-+  OutDataTypeStr=fixdt(1,16,19)
  Backward Taps : Memory  InitialCondition=complex(zeros(numBTaps,1))  InheritSampleTime=on
  Constant2 : Constant  Value=complex(zeros(numBTaps,1))  OutDataTypeStr=fixdt(1,16,4)  SampleTime=-1
  Constant3 : Constant  Value=complex(zeros(numFTaps,1))  OutDataTypeStr=fixdt(1,16,4)  SampleTime=-1
  Decision Buffer : simulink/Discrete/Tapped Delay  vinit=0.0  samptime=-1  NumDelays=numBTaps  DelayOrder=Oldest  includeCurrent=off
  Delay To Reference Tap : Delay  DelayLength=refTap  ExternalReset=Level
      settings: InputPortMap=u0,r5
  Delay To Reference Tap2 : Delay  DelayLength=refTap+1
  Delay data so DFE can reset1 : Delay  DelayLength=1
  Dot Product : DotProduct  OutDataTypeStr=fixdt(1,16,14)  SaturateOnIntegerOverflow=on  InputSameDT=on
  Dot Product1 : DotProduct  OutDataTypeStr=fixdt(1,16,18)  SaturateOnIntegerOverflow=on  InputSameDT=on
  Forward Taps : Memory  InitialCondition=[complex(zeros(numFTaps-1,1));1]  InheritSampleTime=on
  InputBuffer : simulink/Discrete/Tapped Delay  vinit=0.0  samptime=-1  NumDelays=numFTaps  DelayOrder=Oldest  includeCurrent=off
  Map Symbol : Subsystem
  Math Function : Math  Operator=conj  RndMeth=Zero  SaturateOnIntegerOverflow=on
  Pipeline Delay1 : Delay  DelayLength=1
  Pipeline Delay2 : Delay  DelayLength=1
  Product1 : Product  OutDataTypeStr=fixdt(1,16,22)
  Product2 : Product  OutDataTypeStr=fixdt(1,16,22)
  Product3 : Product  OutDataTypeStr=fixdt(1,16,21)
  Reciprocal : Product  Inputs=/  OutDataTypeStr=fixdt(0,16,22)  SaturateOnIntegerOverflow=on  RndMeth=Zero
  Subtract : Sum  Inputs=-+  OutDataTypeStr=fixdt(1,16,15)
  Subtract2 : Sum  Inputs=+-  OutDataTypeStr=fixdt(1,16,14)
  Switch : Switch  Criteria=u2 > Threshold  OutDataTypeStr=fixdt(1,16,15)
  Switch2 : Switch  Criteria=u2 > Threshold  OutDataTypeStr=fixdt(1,16,14)
  eqOut : Outport
  err : Outport  Port=2
  start : Outport  Port=3
  wires:
  InputBuffer/1 -> Product2/2, Dot Product/2
  Dot Product/1 -> Subtract2/1
  Dot Product1/1 -> Subtract2/2
  Subtract2/1 -> Map Symbol/1(In1), Subtract/1, eqOut/1
  Subtract/1 -> Math Function/1
  Math Function/1 -> err/1, Product1/1
  Forward Taps/1 -> Dot Product/1, Add/2
  Map Symbol/1(d) -> Subtract/2, Decision Buffer/1
  reset/1 -> Delay To Reference Tap2/1, Delay data so DFE can reset1/1, [reset], Map Symbol/3(reset)
  EQmu/1 -> Pipeline Delay1/1
  Backward Taps/1 -> Dot Product1/1, Add1/2
  Decision Buffer/1 -> Product3/2, Dot Product1/2
  Add1/1 -> Switch/3
  Switch/1 -> Backward Taps/1
  Constant2/1 -> Switch/1
  [reset] -> Switch/2
  Switch2/1 -> Forward Taps/1
  Add/1 -> Switch2/3
  Constant3/1 -> Switch2/1
  [reset] -> Switch2/2
  Product2/1 -> Add/1
  Product1/1 -> Product2/1, Product3/1
  Product3/1 -> Add1/1
  dataIn/1 -> InputBuffer/1
  training/1 -> Delay To Reference Tap/1
  Delay To Reference Tap/1 -> Map Symbol/2(training)
  Delay data so DFE can reset1/1 -> Delay To Reference Tap/2
  Delay To Reference Tap2/1 -> start/1
  Reciprocal/1 -> Pipeline Delay2/1
  Pipeline Delay2/1 -> Product1/2
  Pipeline Delay1/1 -> Reciprocal/1

== system combinedTxRx_ADIDMA/Combined TX and RX/Receiver HDL/Frame Recover/Equalization and Demodulation/DFE/Packeted To Unpacked ==
  In1 : Inport
  Extract Bits : simulink/Logic and Bit Operations/Extract Bits  bitsToExtract=Range of bits  numBits=8  bitIdxRange=[1]  outScalingMode=Treat bit field as an integer
      settings: SourceProductName=Simulink
  Extract Bits1 : simulink/Logic and Bit Operations/Extract Bits  bitsToExtract=Range of bits  numBits=8  bitIdxRange=[0]  outScalingMode=Treat bit field as an integer
      settings: SourceProductName=Simulink
  Vector Concatenate : Concatenate
  Out1 : Outport
  wires:
  In1/1 -> Extract Bits1/1, Extract Bits/1
  Extract Bits/1 -> Vector Concatenate/1
  Extract Bits1/1 -> Vector Concatenate/2
  Vector Concatenate/1 -> Out1/1

== system combinedTxRx_ADIDMA/Combined TX and RX/Receiver HDL/Frame Recover/Gardner Timing Recovery/Gardner TED Blocks/Imag Error ==
  data : Inport
  strobe sum : Inport  Port=2
  Delay : Delay  DelayLength=1
  Product1 : Product
  Sub : Sum  Inputs=+-
  TED Buffer Update1 : Subsystem
  Out1 : Outport
  wires:
  Product1/1 -> Out1/1
  Sub/1 -> Product1/2
  data/1 -> Sub/2, Delay/1
  strobe sum/1 -> TED Buffer Update1/2(strobe sum)
  TED Buffer Update1/2(oldest) -> Sub/1
  Delay/1 -> TED Buffer Update1/1(new data)
  TED Buffer Update1/1(Middle Indx) -> Product1/1

== system combinedTxRx_ADIDMA/Combined TX and RX/Receiver HDL/Frame Recover/Gardner Timing Recovery/Gardner TED Blocks/Real Error ==
  data : Inport
  strobe sum : Inport  Port=2
  Delay : Delay  DelayLength=1
  Product1 : Product  OutDataTypeStr=fixdt(1,16,12)
  Sub : Sum  Inputs=+-
  TED Buffer Update1 : Subsystem
  Out1 : Outport
  wires:
  Product1/1 -> Out1/1
  Sub/1 -> Product1/2
  data/1 -> Sub/2, Delay/1
  strobe sum/1 -> TED Buffer Update1/2(strobe sum)
  TED Buffer Update1/2(oldest) -> Sub/1
  Delay/1 -> TED Buffer Update1/1(new data)
  TED Buffer Update1/1(Middle Indx) -> Product1/1

== system combinedTxRx_ADIDMA/Combined TX and RX/Receiver HDL/Frame Recover/Gardner Timing Recovery/InterpControl_Blocks1/Calculate New mu ==
  note: Good at fixd(0,16,12)
  W : Inport
  NCOCounter : Inport  Port=2
  Math Reciprocal : Math  Operator=reciprocal  OutDataTypeStr=fixdt(1,16,12)  RndMeth=Zero  SaturateOnIntegerOverflow=on
  Product : Product  OutDataTypeStr=fixdt(0,15,14)
  mu : Outport
  wires:
  Product/1 -> mu/1
  Math Reciprocal/1 -> Product/1
  NCOCounter/1 -> Product/2
  W/1 -> Math Reciprocal/1

== system combinedTxRx_ADIDMA/Combined TX and RX/Receiver HDL/Frame Recover/Gardner Timing Recovery/InterpControl_Blocks1/Mod 1 ==
  In1 : Inport
  Add : Sum
  Compare To Constant : simulink/Logic and Bit Operations/Compare To Constant  relop=<  const=1  OutDataTypeStr=boolean
  Compare To Constant1 : simulink/Logic and Bit Operations/Compare To Constant  relop=>=  const=0  OutDataTypeStr=boolean
  Constant : Constant  OutDataTypeStr=fixdt(0,1,0)  SampleTime=-1
  Constant1 : Constant  OutDataTypeStr=fixdt(0,1,0)  SampleTime=-1
  Logical Operator : Logic  AllPortsSameDT=off  OutDataTypeStr=boolean
  Subtract : Sum  Inputs=+-
  Switch : Switch  Criteria=u2 > Threshold
  Switch1 : Switch
  Out1 : Outport
  wires:
  Switch/1 -> Out1/1
  Constant/1 -> Subtract/2
  Constant1/1 -> Add/2
  Switch1/1 -> Switch/3
  Subtract/1 -> Switch1/1
  Add/1 -> Switch1/3
  In1/1 -> Switch1/2, Compare To Constant1/1, Compare To Constant/1, Switch/1, Add/1, Subtract/1
  Compare To Constant1/1 -> Logical Operator/1
  Compare To Constant/1 -> Logical Operator/2
  Logical Operator/1 -> Switch/2

== system combinedTxRx_ADIDMA/Combined TX and RX/Transmitter HDL/Transmitter HDL/Packet Generation/Payload/Enable Latch ==
  note: This block will latch when start flag is high and then latch low when end flag arrives
  mode : Inport
  start : Inport  Port=2
  end : Inport  Port=3
  Compare To Constant : simulink/Logic and Bit Operations/Compare To Constant  relop=>=  const=uint8(1)  OutDataTypeStr=boolean
  Compare To Constant1 : simulink/Logic and Bit Operations/Compare To Constant  relop===  const=uint8(1)  OutDataTypeStr=boolean
  HDL Counter1 : hdlsllib/Sources/HDL Counter  CountType=Count limited  CountInit=0  CountStep=1  CountMax=1  CountFromType=Initial value  CountFrom=0  CountResetPort=on  CountLoadPort=off  CountEnbPort=on  CountDirPort=off  CountDataType=Unsigned  CountWordLen=8  CountFracLen=0  CountSampTime=1
      settings: SourceProductBaseCode=HD
  Logical Operator : Logic  AllPortsSameDT=off  OutDataTypeStr=boolean
  Logical Operator1 : Logic  AllPortsSameDT=off  OutDataTypeStr=boolean
  Logical Operator2 : Logic  Operator=OR  AllPortsSameDT=off  OutDataTypeStr=boolean
  MATLAB Function : MATLAB Function  Commented=on  TreatAsAtomicUnit=on
  Terminator : Terminator  Commented=on
  valid : Outport
  wires:
  mode/1 -> Compare To Constant/1
  Compare To Constant/1 -> Logical Operator1/1, Logical Operator/1
  start/1 -> MATLAB Function/1(startpacket), Logical Operator/2
  end/1 -> MATLAB Function/2(endpacket), Logical Operator1/2
  HDL Counter1/1 -> Compare To Constant1/1
  Logical Operator1/1 -> HDL Counter1/1
  Logical Operator/1 -> Logical Operator2/1, HDL Counter1/2
  Compare To Constant1/1 -> Logical Operator2/2
  MATLAB Function/1(outEnable) -> Terminator/1
  Logical Operator2/1 -> valid/1

== system combinedTxRx_ADIDMA/Combined TX and RX/Transmitter HDL/Transmitter HDL/Packet Generation/Payload/HDL Scrambler 2 bits ==
  bitsIn : Inport
  reset : Inport  Port=2
  Buffer Manage : MATLAB Function  TreatAsAtomicUnit=on
  Delay : Delay  DelayLength=1  InitialCondition=false
  Delay1 : Delay  DelayLength=1  InitialCondition=false
  Demux : Demux  Outputs=2
  Display1 : Display
  Display3 : Display
  Mux : Mux  Inputs=2
  Mux1 : Mux  Inputs=2
  Selector : Selector  IndexOptions=Index vector (dialog)  Indices=find(poly(2:end))  OutputSizes=1
  Selector1 : Selector  IndexOptions=Index vector (dialog)  Indices=1+find(poly(2:end))  OutputSizes=1
  state_xor1 : Logic  Operator=XOR  IconShape=distinctive  AllPortsSameDT=off  OutDataTypeStr=boolean
  state_xor2 : Logic  Operator=XOR  Inputs=1  IconShape=distinctive  AllPortsSameDT=off  OutDataTypeStr=boolean
  state_xor3 : Logic  Operator=XOR  Inputs=1  IconShape=distinctive  AllPortsSameDT=off  OutDataTypeStr=boolean
  state_xor4 : Logic  Operator=XOR  IconShape=distinctive  AllPortsSameDT=off  OutDataTypeStr=boolean
  bitsOut : Outport
  wires:
  bitsIn/1 -> Display1/1, Demux/1
  Selector/1 -> state_xor2/1
  state_xor2/1 -> Display3/1, state_xor1/1
  Demux/1 -> state_xor1/2
  state_xor1/1 -> Mux1/2, Mux/1, Delay/1
  Mux/1 -> bitsOut/1
  Mux1/1 -> Selector1/1
  Buffer Manage/1(outBuffer) -> Mux1/1, Selector/1
  Selector1/1 -> state_xor3/1
  state_xor3/1 -> state_xor4/1
  Demux/2 -> state_xor4/2
  state_xor4/1 -> Delay1/1, Mux/2
  Delay/1 -> Buffer Manage/1(bit1)
  reset/1 -> Buffer Manage/3(reset)
  Delay1/1 -> Buffer Manage/2(bit2)

== system combinedTxRx_ADIDMA/Combined TX and RX/Transmitter HDL/Transmitter HDL/Packet Generation/Preamble/Unpack1 ==
  In1 : Inport
  Data Type Conversion : DataTypeConversion  OutDataTypeStr=boolean
  Extract Bits : simulink/Logic and Bit Operations/Extract Bits  bitsToExtract=Range of bits  numBits=8  bitIdxRange=[1]  outScalingMode=Treat bit field as an integer
      settings: SourceProductName=Simulink
  Extract Bits1 : simulink/Logic and Bit Operations/Extract Bits  bitsToExtract=Range of bits  numBits=8  bitIdxRange=[0]  outScalingMode=Treat bit field as an integer
      settings: SourceProductName=Simulink
  Vector Concatenate : Concatenate
  Out1 : Outport
  wires:
  In1/1 -> Extract Bits1/1, Extract Bits/1
  Extract Bits/1 -> Vector Concatenate/1
  Extract Bits1/1 -> Vector Concatenate/2
  Vector Concatenate/1 -> Data Type Conversion/1
  Data Type Conversion/1 -> Out1/1

== system combinedTxRx_ADIDMA/Combined TX and RX/Transmitter HDL/Transmitter HDL/Packet Generation/Random Data/Unpack ==
  In1 : Inport
  Data Type Conversion : DataTypeConversion  OutDataTypeStr=boolean
  Extract Bits : simulink/Logic and Bit Operations/Extract Bits  bitsToExtract=Range of bits  numBits=8  bitIdxRange=[0]  outScalingMode=Treat bit field as an integer
      settings: SourceProductName=Simulink
  Extract Bits1 : simulink/Logic and Bit Operations/Extract Bits  bitsToExtract=Range of bits  numBits=8  bitIdxRange=[1]  outScalingMode=Treat bit field as an integer
      settings: SourceProductName=Simulink
  Vector Concatenate : Concatenate
  Out1 : Outport
  wires:
  In1/1 -> Extract Bits1/1, Extract Bits/1
  Extract Bits/1 -> Vector Concatenate/1
  Extract Bits1/1 -> Vector Concatenate/2
  Vector Concatenate/1 -> Data Type Conversion/1
  Data Type Conversion/1 -> Out1/1

== system combinedTxRx_ADIDMA/Combined TX and RX/Receiver HDL/Frame Recover/Equalization and Demodulation/DFE/DFE/Map Symbol ==
  In1 : Inport  OutDataTypeStr=fixdt(1,16,14)
  training : Inport  Port=2  OutDataTypeStr=fixdt(1,16,15)
  reset : Inport  Port=3
  Decision Directed : Subsystem
  Delay : Delay  DelayLength=1
  HDL Counter : hdlsllib/Sources/HDL Counter  CountType=Count limited  CountInit=0  CountStep=1  CountMax=2^18  CountFromType=Initial value  CountFrom=0  CountResetPort=on  CountLoadPort=off  CountEnbPort=off  CountDirPort=off  CountDataType=Unsigned  CountWordLen=32  CountFracLen=0  CountSampTime=1
      settings: SourceProductBaseCode=HD
  Switch : Switch  Criteria=u2 > Threshold  Threshold=numTrainingSamples  OutDataTypeStr=fixdt(1,16,15)
  d : Outport
  wires:
  In1/1 -> Decision Directed/1(eqOut)
  Switch/1 -> d/1
  reset/1 -> HDL Counter/1
  HDL Counter/1 -> Switch/2
  Decision Directed/1(decision) -> Switch/1
  training/1 -> Delay/1
  Delay/1 -> Switch/3

== system combinedTxRx_ADIDMA/Combined TX and RX/Receiver HDL/Frame Recover/Gardner Timing Recovery/Gardner TED Blocks/Imag Error/TED Buffer Update1 ==
  new data : Inport
  strobe sum : Inport  Port=2
  Delay{,1..3} (4 alike) : Delay  DelayLength=1
  Multiport Switch{,1..3} (4 alike) : MultiPortSwitch  DataPortOrder=Zero-based contiguous  DataPortIndices={0,1,[2,3]}
  Zero bit : Constant  Value=0  OutDataTypeStr=fixdt(1,16,13)  SampleTime=1/RadioSampleRate
  Middle Indx : Outport
  oldest : Outport  Port=2
  wires:
  strobe sum/1 -> Multiport Switch3/1, Multiport Switch2/1, Multiport Switch1/1, Multiport Switch/1
  Delay/1 -> Multiport Switch/2
  Delay1/1 -> Multiport Switch/3, Multiport Switch1/2
  Delay2/1 -> Multiport Switch/4, Multiport Switch1/3, Multiport Switch2/2
  new data/1 -> Multiport Switch3/4, Multiport Switch3/3
  Zero bit/1 -> Multiport Switch2/4
  Delay3/1 -> Multiport Switch1/4, Multiport Switch2/3, Multiport Switch3/2
  Multiport Switch1/1 -> Delay1/1
  Multiport Switch2/1 -> Middle Indx/1, Delay2/1
  Multiport Switch3/1 -> Delay3/1
  Multiport Switch/1 -> Delay/1, oldest/1

== system combinedTxRx_ADIDMA/Combined TX and RX/Receiver HDL/Frame Recover/Gardner Timing Recovery/Gardner TED Blocks/Real Error/TED Buffer Update1 ==
  new data : Inport
  strobe sum : Inport  Port=2
  Delay{,1..3} (4 alike) : Delay  DelayLength=1
  Multiport Switch{,1..3} (4 alike) : MultiPortSwitch  DataPortOrder=Zero-based contiguous  DataPortIndices={0,1,[2,3]}
  Zero bit : Constant  Value=0  OutDataTypeStr=fixdt(1,16,13)  SampleTime=1/RadioSampleRate
  Middle Indx : Outport
  oldest : Outport  Port=2
  wires:
  strobe sum/1 -> Multiport Switch3/1, Multiport Switch2/1, Multiport Switch1/1, Multiport Switch/1
  Delay/1 -> Multiport Switch/2
  Delay1/1 -> Multiport Switch/3, Multiport Switch1/2
  Delay2/1 -> Multiport Switch/4, Multiport Switch1/3, Multiport Switch2/2
  new data/1 -> Multiport Switch3/4, Multiport Switch3/3
  Zero bit/1 -> Multiport Switch2/4
  Delay3/1 -> Multiport Switch1/4, Multiport Switch2/3, Multiport Switch3/2
  Multiport Switch1/1 -> Delay1/1
  Multiport Switch2/1 -> Middle Indx/1, Delay2/1
  Multiport Switch3/1 -> Delay3/1
  Multiport Switch/1 -> Delay/1, oldest/1
